simulink model "furuta_pen_sim"  (R2017a)
settings: Solver=VariableStepAuto  StartTime=0.0  StopTime=10.0  RelTol=1e-3
values from neighbouring files (symbols this model uses):
  anpha_0 = 5    [ANN_params.m]    (also in furuta.m)
  beta0 = 5.8*10^(-4)    (= 0.00058)    [ANN_params.m]    (also in furuta.m)
  beta1 = 1.4142*10^(-3)    (= 0.0014142)    [ANN_params.m]    (also in furuta.m)
  g = 9.81    [ANN_params.m]    (also in furuta.m)
  J0 = 4.4*10^(-3)    (= 0.0044)    [ANN_params.m]    (also in furuta.m)
  J1 = 5.5026*10^(-4)    (= 0.00055026)    [ANN_params.m]    (also in furuta.m)
  ksw = 30    [furuta.m]
  L0 = 0.157    [ANN_params.m]    (also in furuta.m)
  L1 = 0.133    [ANN_params.m]    (also in furuta.m)
  m1 = 0.078    [ANN_params.m]    (also in furuta.m = 0.0933)
  R = 8.53*eye(8)    [ANN_params.m]    (also in furuta.m = [-0.2500,20.6329,-0.6179,2.5406])
  theta_0 = 0    [ANN_params.m]    (also in furuta.m)
  up = 1    [furuta.m]
settings Model: Creator=Chechao  LastModifiedBy=chech
settings ExplorerConfigSet: InternalSimMechanicsExplorerSettings="<ExplorerConfiguration><canonicalview>planar_xy</canonicalview><AnimationSetting><BasePlaybackSpeed>1.0</BasePlaybackSpeed><PlaybackSpeedFactor>1.0</PlaybackSpeedFactor></AnimationSetting><TilePanel><TileInfo><Tiles Columns=\"1\" Count=\"1\" Rows=\"1\"><Column Left=\"2\" Weight=\"1\"/><Column Left=\"815\"/><Row Top=\"2\" Weight=\"1\"/><Row Top=\"278\"/><Tile Height=\"1\" Width=\"1\" X=\"0\" Y=\"0\"/></Tiles></TileInfo><SceneInfo><SceneViewer><BGColor><R>0.60000002384185791</R><G>0.60000002384185791</G><B>0.60000002384185791</B></BGColor><Camera><DoPerspective>off</DoPerspective><Position><X>3.0348189574883895</X><Y>0.89503316987109838</Y><Z>1.1148954709131602</Z></Position><Center><X>1.4216968578267744</X><Y>0.23812580067611089</Y><Z>-0.36954855728247171</Z></Center><Up><X>-0.074382553953715444</X><Y>0.93933115277276391</Y><Z>-0.3348495499443197</Z></Up><ViewLimDist>1</ViewLimDist><YLim>1.1431212443461942</YLim><XLim>3.4422077919638205</XLim></Camera></SceneViewer></SceneInfo></TilePanel><MechEditorPanel><Cameras/><GfxPanelCameraMap/><VideoCreator><PlaybackSpeedRatio>1.0</PlaybackSpeedRatio><FrameRate>30</FrameRate><VideoFormat>Motion JPEG AVI</VideoFormat><FrameSize>auto</FrameSize></VideoCreator></MechEditorPanel></ExplorerConfiguration>"

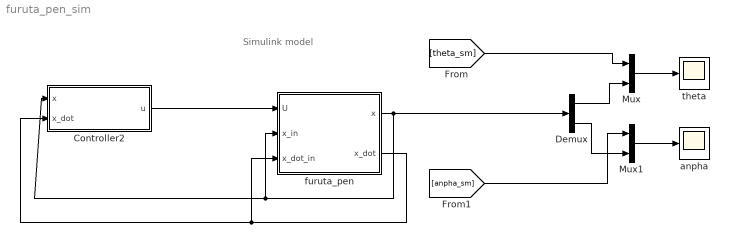
== system furuta_pen_sim ==
  note: Simulink model
  Controller2 : Subsystem
  Demux : Demux  Outputs=2
  Mux : Mux  Inputs=2
  Mux1 : Mux  Inputs=2
  anpha : Scope
  furuta_pen : Subsystem
  theta : Scope
  wires:
  furuta_pen/2(x_dot) -> Controller2/2(x_dot), furuta_pen/3(x_dot_in)
  furuta_pen/1(x) -> Demux/1, Controller2/1(x), furuta_pen/2(x_in)
  Controller2/1(u) -> furuta_pen/1(U)
  Demux/1 -> Mux/2
  Mux/1 -> theta/1
  Mux1/1 -> anpha/1
  [theta_sm] -> Mux/1
  [anpha_sm] -> Mux1/1
  Demux/2 -> Mux1/2

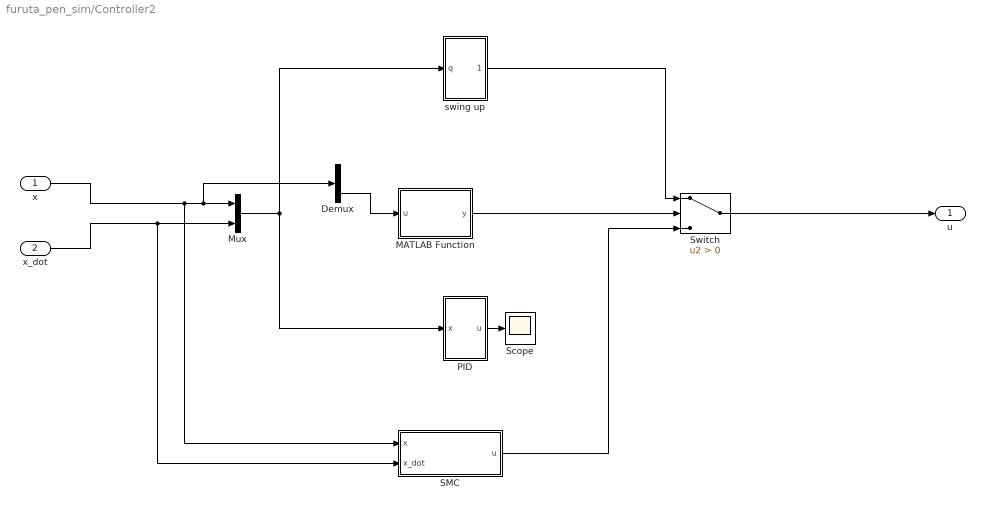
== system furuta_pen_sim/Controller2 ==
  x : Inport
  x_dot : Inport  Port=2
  Demux : Demux  Outputs=2
  MATLAB Function : MATLAB Function  TreatAsAtomicUnit=on
  Mux : Mux  Inputs=2
  PID : Subsystem
  SMC : Subsystem
  Scope : Scope
  Switch : Switch  Criteria=u2 > Threshold
  swing up : Subsystem
  u : Outport
  wires:
  x/1 -> SMC/1(x), Demux/1, Mux/1
  x_dot/1 -> SMC/2(x_dot), Mux/2
  Mux/1 -> PID/1(x), swing up/1(q)
  Switch/1 -> u/1
  swing up/1(Out1) -> Switch/1
  MATLAB Function/1(y) -> Switch/2
  Demux/2 -> MATLAB Function/1(u)
  PID/1(u) -> Scope/1
  SMC/1(u) -> Switch/3

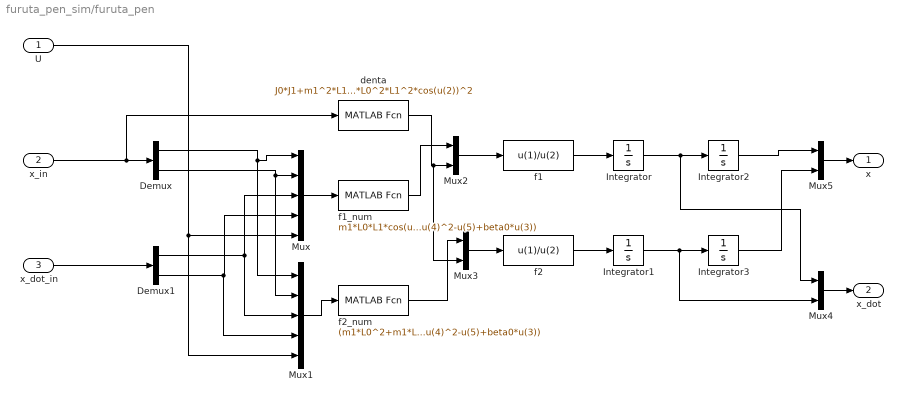
== system furuta_pen_sim/furuta_pen ==
  U : Inport
  x_in : Inport  Port=2
  x_dot_in : Inport  Port=3
  Demux : Demux  Outputs=2
  Demux1 : Demux  Outputs=2
  Integrator : Integrator
  Integrator1 : Integrator
  Integrator2 : Integrator  InitialCondition=theta_0*pi/180
  Integrator3 : Integrator  InitialCondition=anpha_0/180*pi
  Mux : Mux  Inputs=5
  Mux1 : Mux  Inputs=5
  Mux{2..5} (4 alike) : Mux  Inputs=2
  denta : MATLABFcn  MATLABFcn=J0*J1+m1^2*L1^4*sin(u(2))^2+m1^2*L0^2*L1^2+J0*m1*L1^2+J1*m1*L0^2+J1*m1*L1^2*sin(u(2))^2-m1^2*L0^2*L1^2*cos(u(2))^2
  f1 : MATLABFcn  MATLABFcn=u(1)/u(2)
  f1_num : MATLABFcn  MATLABFcn=m1*L0*L1*cos(u(2))*(0.5*m1*L1^2*sin(2*u(2))*u(3)^2+m1*g*L1*sin(u(2))-beta1*u(4))-(m1*L1^2+J1)*(m1*L1^2*sin(2*u(2))*u(3)*u(4)+m1*L0*L1*sin(u(2))*u(4)^2-u(5)+beta0*u(3))
  f2 : MATLABFcn  MATLABFcn=u(1)/u(2)
  f2_num : MATLABFcn  MATLABFcn=(m1*L0^2+m1*L1^2*sin(u(2))^2+J0)*(0.5*m1*L1^2*sin(2*u(2))*u(3)^2+m1*g*L1*sin(u(2))-beta1*u(4))-m1*L0*L1*cos(u(2))*(m1*L1^2*sin(2*u(2))*u(3)*u(4)+m1*L0*L1*sin(u(2))*u(4)^2-u(5)+beta0*u(3))
  x : Outport
  x_dot : Outport  Port=2
  wires:
  x_in/1 -> Demux/1, denta/1
  Mux/1 -> f1_num/1
  Mux1/1 -> f2_num/1
  Mux2/1 -> f1/1
  denta/1 -> Mux3/2, Mux2/2
  f1_num/1 -> Mux2/1
  Mux3/1 -> f2/1
  f2_num/1 -> Mux3/1
  f1/1 -> Integrator/1
  f2/1 -> Integrator1/1
  Integrator/1 -> Mux4/1, Integrator2/1
  Integrator1/1 -> Mux4/2, Integrator3/1
  Mux4/1 -> x_dot/1
  Mux5/1 -> x/1
  Integrator2/1 -> Mux5/1
  Integrator3/1 -> Mux5/2
  U/1 -> Mux1/5, Mux/5
  x_dot_in/1 -> Demux1/1
  Demux/1 -> Mux1/1, Mux/1
  Demux/2 -> Mux1/2, Mux/2
  Demux1/2 -> Mux1/4, Mux/4
  Demux1/1 -> Mux1/3, Mux/3

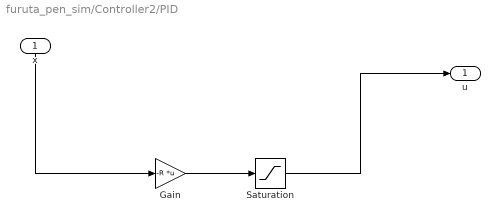
== system furuta_pen_sim/Controller2/PID ==
  x : Inport
  Gain : Gain  Gain=-R  Multiplication=Matrix(K*u)
  Saturation : Saturate  UpperLimit=up  LowerLimit=-up
  u : Outport
  wires:
  Saturation/1 -> u/1
  x/1 -> Gain/1
  Gain/1 -> Saturation/1

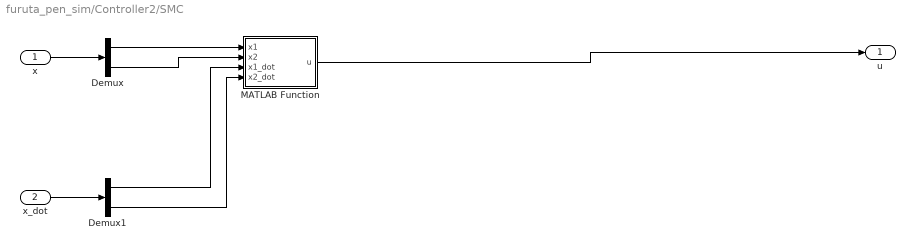
== system furuta_pen_sim/Controller2/SMC ==
  x : Inport
  x_dot : Inport  Port=2
  Demux : Demux  Outputs=2
  Demux1 : Demux  Outputs=2
  MATLAB Function : MATLAB Function  TreatAsAtomicUnit=on
  u : Outport
  wires:
  MATLAB Function/1(u) -> u/1
  x/1 -> Demux/1
  Demux/1 -> MATLAB Function/1(x1)
  Demux/2 -> MATLAB Function/2(x2)
  Demux1/1 -> MATLAB Function/3(x1_dot)
  Demux1/2 -> MATLAB Function/4(x2_dot)
  x_dot/1 -> Demux1/1

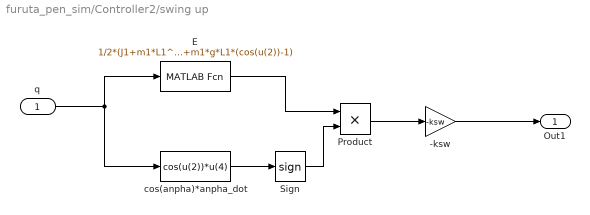
== system furuta_pen_sim/Controller2/swing up ==
  q : Inport
  -ksw : Gain  Gain=-ksw
  E : MATLABFcn  MATLABFcn=1/2*(J1+m1*L1^2)*u(4)^2+m1*g*L1*(cos(u(2))-1)
  Product : Product
  Sign : Signum
  cos(anpha)*anpha_dot : MATLABFcn  MATLABFcn=cos(u(2))*u(4)
  Out1 : Outport
  wires:
  Sign/1 -> Product/2
  E/1 -> Product/1
  Product/1 -> -ksw/1
  cos(anpha)*anpha_dot/1 -> Sign/1
  q/1 -> E/1, cos(anpha)*anpha_dot/1
  -ksw/1 -> Out1/1

== matlab function furuta_pen_sim/Controller2/MATLAB Function ==
  data: u input; y output
function y = fcn(u)
if abs(u)<20*pi/180
    y = 0;
else
    y= 1;
end

== matlab function furuta_pen_sim/Controller2/SMC/MATLAB Function ==
  data: x1 input; u output; x2 input; x1_dot input; x2_dot input
function u = fcn(x1,x2,x1_dot,x2_dot)
b = [14.8452;12.5278];
C = [0,17.3564;
    0,67.377];
D = [-0.1172,-0.2411;
    -0.0989,-0.09359];
M = [0.5,0;
    0,10];
Q= [5/16,-3/4;
    -3/4,9/4];
R = [161/160 -3;
    -3 9];
x = [x1;x2];
x_dot = [x1_dot;x2_dot];
s = M*x+x_dot;
u = -(s'*R*s+s'*Q*(M+D)*x_dot+s'*Q*C*x)/(s'*Q*b);
